simulink model "IndirectFOCControl"  (R2022b)
settings: Solver=VariableStepAuto  StartTime=0.0  StopTime=1  RelTol=1e-3
InitFcn:
  | Data
values from neighbouring files (symbols this model uses):
  delta = 10e-3    (= 0.01)    [Data.m]
  p = 6    [Data.m]    (also in FOC_BANG_Script.m; IFOCdatav6.m)
  Tr = Lm*(1+sigma_r)/Rr    [FOC_BANG_Script.m]    (also in IFOCdatav6.m)
  Vdc = 350    [Data.m]    (also in FOC_BANG_Script.m; IFOCdatav6.m)
libraries: spsControlledVoltageSourceLib x3, spsCurrentMeasurementLib x3, spsAsynchronousMachineSIUnitsLib x1, slpidlib x1, spspowerguiLib x1
settings Model: Creator=v4pal  LastModifiedBy=v4pal

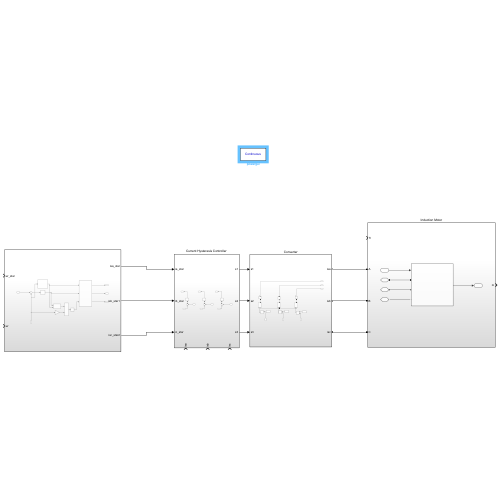
[thumbnail: Simulink's stored preview of the top-level diagram]
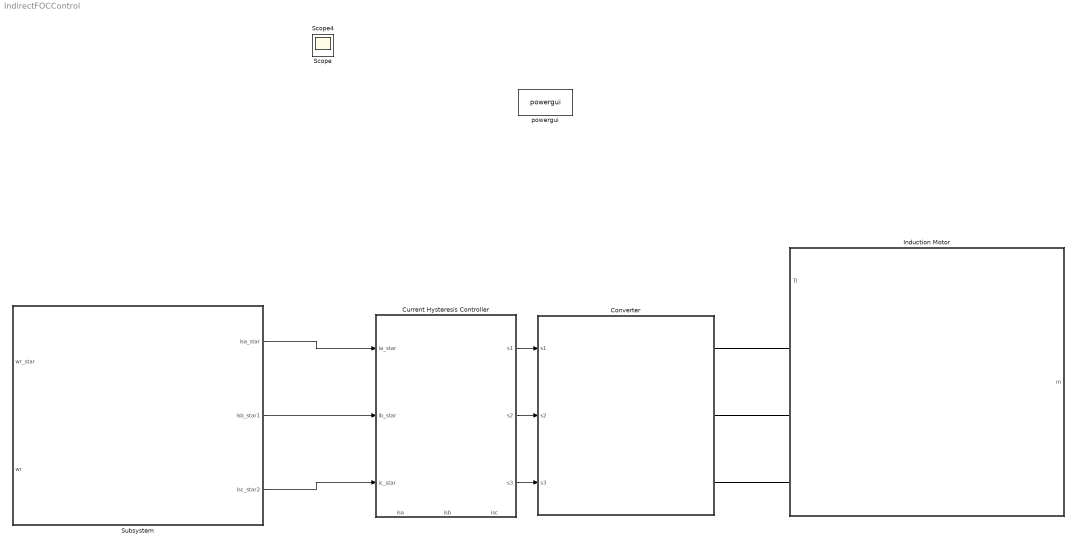
== system IndirectFOCControl ==
  Converter : Subsystem
  "Current Hysteresis Controller " : Subsystem
      settings: PortSchema="{\"entries\":[{\"content\":{\"sides\":[{\"content\":{\"connectorIds\":[\"In1\",\"In2\",\"In3\"]},\"type\":\"ConnectorPlacement.EquallySpacedRectSide\",\"uuid\":\"0262a758-344e-4b59-aa8e-2379075e1762\"},{\"content\":{\"connectorIds\":[\"Out1\",\"Out2\",\"Out3\"],\"side\":\"RIGHT\"},\"type\":\"ConnectorPlacement.EquallySpacedRectSide\",\"uuid\":\"0941517e-4382-4a35-83ac-77ea733cd1ec\"},{\"content\":{\"connectorIds\":[],\"side\":\"TOP\"},\"type\":\"ConnectorPlacement.EquallySpacedRectSide\",\"uuid\":\"ef1a3383-760d-4746-8858-884eb9913812\"},{\"content\":{\"connectorIds\":[\"In4\",\"In5\",\"In6\"],\"side\":\"BOTTOM\"},\"type\":\"ConnectorPlacement.EquallySpacedRectSide\",\"uuid\":\"40fa37ed-c9f4-4172-881b-821ac55ca797\"}]},\"type\":\"ConnectorPlacement.EquallySpacedConnector\",\"uuid\":\"06b611ca-38e4-4d8c-842f-a6960a505aa4\"}],\"packageUris\":[\"http://schema.mathworks.com/mf0/Connector/R2020b\"],\"version\":\"1.0\"}"
  Induction Motor : Subsystem
  Subsystem : Subsystem
  powergui : spspowerguiLib/powergui  Priority=1  SimulationMode=Continuous  SampleTime=50e-6  frequency=60  Iterations=50  frequencyindice=0  Pbase=100e6  ErrMax=1e-4  UnitsV=kV  UnitsW=MW  buscounter=0  FunctionMessages=off  echomessages=off  EnableUseOfTLC=off  CurrentSourceSwitches=off  DisableSnubberDevices=off  DisableRonSwitches=off  DisableVfSwitches=off  DisplayEquations=off  AutomaticDiscreteSolvers=off  SolverType=Tustin/Backward Euler (TBE)  Interpol=off  ExternalGateDelay=off  methode=off  Ts=100  x0status=blocks  SPID=on  SwTol=0  HookPort=off  NonlinearTolerance=1e-4  nMaxIteration=100  ContinueOnMaxIteration=off  RestoreLinks=warning  ResistiveCurrentMeasurement=off  Frange=[0:2:500]  Ylog=off  Xlog=on  ShowGrid=off  save=off  variable=ZData  structure=0  ZoomFFT=off  StartTime=0.0  cycles=1  DisplayStyle=1  fundamental=60  FreqAxis=off  MaxFrequency=1000  frequencyindicesteady=1  RmsSteady=1  display=off
  Scope : Scope
  Scope4 : Scope
  wires:
  "Current Hysteresis Controller "/1(s1) -> Converter/1(s1)
  "Current Hysteresis Controller "/2(s2) -> Converter/2(s2)
  "Current Hysteresis Controller "/3(s3) -> Converter/3(s3)
  Subsystem/1(isa_star) -> "Current Hysteresis Controller "/1(ia_star)
  Subsystem/2(isb_star1) -> "Current Hysteresis Controller "/2(ib_star)
  Subsystem/3(isc_star2) -> "Current Hysteresis Controller "/3(ic_star)
  connections:
  Induction Motor/LConn1 -- Converter/RConn1
  Converter/RConn2 -- Induction Motor/LConn2
  Induction Motor/LConn3 -- Converter/RConn3

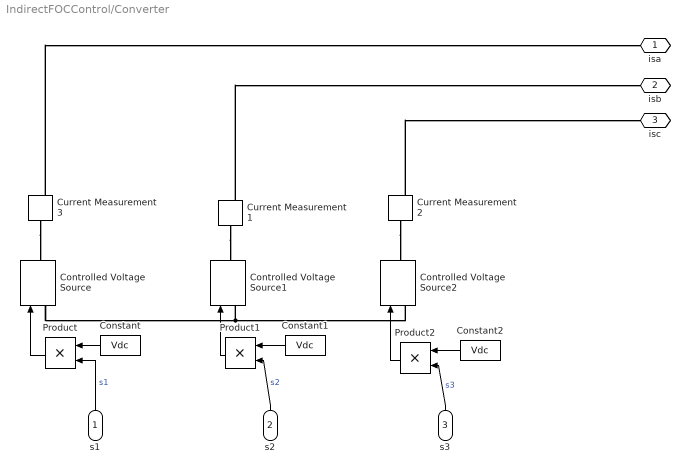
== system IndirectFOCControl/Converter ==
  s1 : Inport
  s2 : Inport  Port=2
  s3 : Inport  Port=3
  Constant : Constant  Value=Vdc
  Constant1 : Constant  Value=Vdc
  Constant2 : Constant  Value=Vdc
  Controlled Voltage Source : spsControlledVoltageSourceLib/Controlled Voltage Source  Initialize=on  Source_Type=AC  Amplitude=0  Phase=0  Frequency=0  Measurements=None
  Controlled Voltage Source1 : spsControlledVoltageSourceLib/Controlled Voltage Source  Initialize=on  Source_Type=AC  Amplitude=0  Phase=0  Frequency=0  Measurements=None
  Controlled Voltage Source2 : spsControlledVoltageSourceLib/Controlled Voltage Source  Initialize=on  Source_Type=AC  Amplitude=0  Phase=0  Frequency=0  Measurements=None
  Current Measurement1 : spsCurrentMeasurementLib/Current Measurement  PhasorSimulation=off  OutputType=Complex  PSBequivalent=0
  Current Measurement2 : spsCurrentMeasurementLib/Current Measurement  PhasorSimulation=off  OutputType=Complex  PSBequivalent=0
  Current Measurement3 : spsCurrentMeasurementLib/Current Measurement  PhasorSimulation=off  OutputType=Complex  PSBequivalent=0
  Product : Product
  Product1 : Product
  Product2 : Product
  isa : PMIOPort  Side=Right
  isb : PMIOPort  Port=2  Side=Right
  isc : PMIOPort  Port=3  Side=Right
  wires:
  Product2/1 -> Controlled Voltage Source2/1
  Constant2/1 -> Product2/1
  Constant/1 -> Product/1
  Product1/1 -> Controlled Voltage Source1/1
  Product/1 -> Controlled Voltage Source/1
  Constant1/1 -> Product1/1
  s2/1 -> Product1/2  "s2"
  s1/1 -> Product/2  "s1"
  s3/1 -> Product2/2  "s3"
  connections:
  Current Measurement1/LConn1 -- Controlled Voltage Source1/RConn1
  Controlled Voltage Source/LConn1 -- Controlled Voltage Source2/LConn1 -- Controlled Voltage Source1/LConn1
  Current Measurement3/LConn1 -- Controlled Voltage Source/RConn1
  Current Measurement2/RConn1 -- isc/RConn1
  Current Measurement2/LConn1 -- Controlled Voltage Source2/RConn1
  Current Measurement1/RConn1 -- isb/RConn1
  Current Measurement3/RConn1 -- isa/RConn1

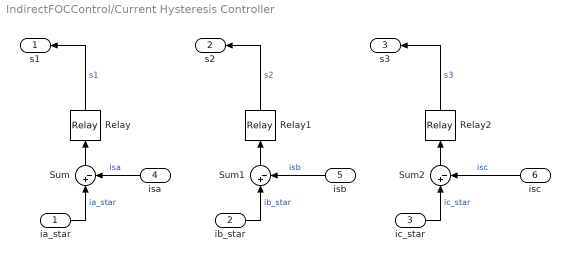
== system IndirectFOCControl/Current Hysteresis Controller  ==
  ia_star : Inport
  ib_star : Inport  Port=2
  ic_star : Inport  Port=3
  isa : Inport  Port=4
  isb : Inport  Port=5
  isc : Inport  Port=6
  Relay : Relay  OnSwitchValue=delta  OffSwitchValue=0
  Relay1 : Relay  OnSwitchValue=delta  OffSwitchValue=0
  Relay2 : Relay  OnSwitchValue=delta  OffSwitchValue=0
  Sum : Sum  Inputs=|+-
  Sum1 : Sum  Inputs=|+-
  Sum2 : Sum  Inputs=|+-
  s1 : Outport
  s2 : Outport  Port=2
  s3 : Outport  Port=3
  wires:
  Sum/1 -> Relay/1
  Sum2/1 -> Relay2/1
  ia_star/1 -> Sum/1  "ia_star"
  isc/1 -> Sum2/2  "isc"
  ic_star/1 -> Sum2/1  "ic_star"
  isa/1 -> Sum/2  "isa"
  Sum1/1 -> Relay1/1
  ib_star/1 -> Sum1/1  "ib_star"
  isb/1 -> Sum1/2  "isb"
  Relay2/1 -> s3/1  "s3"
  Relay/1 -> s1/1  "s1"
  Relay1/1 -> s2/1  "s2"

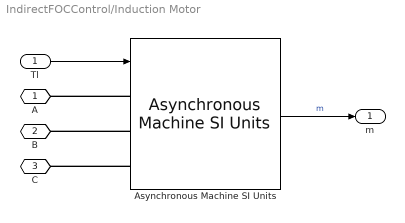
== system IndirectFOCControl/Induction Motor ==
  Tl : Inport
  Asynchronous Machine SI Units : spsAsynchronousMachineSIUnitsLib/Asynchronous Machine SI Units  RotorType=Squirrel-cage  PresetModel=No  MechanicalLoad=Torque Tm  ShowDetailedParameters=on  ReferenceFrame=Rotor  Units=SI  MeasurementBus=off  NominalParameters=[1.845e+04 400 50]  VoltageRatio=1  Stator=[0.5968 0.0003495]  Rotor=[0.6258 0.005473]  Cage1=[0.4155 0.002066]  Cage2=[0.4168 0.0003495]  Lm=0.0354  Mechanical=[0.05 0.005879 2]  PolePairs=2  InitialConditions=[0 0 0 0 0 0 0 0]  SimulateSaturation=off  Saturation=[14.03593122, 27.81365428, 53.79336849, 72.68890987, 97.98006896, 148.6815601, 215.7428561, 302.9841135, 428.7778367 ; 230, 322, 414, 460, 506, 552, 598, 644, 690]  LoadFlowParameters=1492000  TsPowergui=0  TsBlock=-1  IterativeModel=Trapezoidal non iterative  IterativeDiscreteModel=Trapezoidal non iterative  Pmec=1.492e+006
  A : PMIOPort  Side=Left
  B : PMIOPort  Port=2  Side=Left
  C : PMIOPort  Port=3  Side=Left
  m : Outport
  wires:
  Tl/1 -> Asynchronous Machine SI Units/1
  Asynchronous Machine SI Units/1 -> m/1  "m"
  connections:
  Asynchronous Machine SI Units/LConn3 -- C/RConn1
  Asynchronous Machine SI Units/LConn2 -- B/RConn1
  Asynchronous Machine SI Units/LConn1 -- A/RConn1

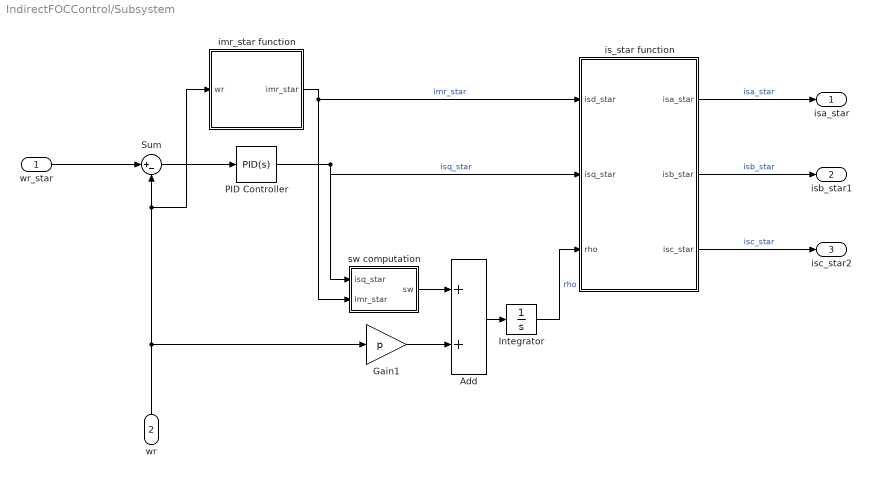
== system IndirectFOCControl/Subsystem ==
  wr_star : Inport
  wr : Inport  Port=2
  Add : Sum
  Gain1 : Gain  Gain=p
  Integrator : Integrator
  PID Controller : slpidlib/PID Controller  Controller=PID  Form=Parallel  TimeDomain=Continuous-time  UseExternalTs=off  SampleTime=-1  IntegratorMethod=Forward Euler  FilterMethod=Forward Euler  ControllerParametersSource=internal  P=1  I=1  UseKiTs=off  D=0  N=100  UseFilter=on  TunerSelectOption=Transfer Function Based (PID Tuner App)  InitialConditionSource=internal  InitialConditionForIntegrator=0  InitialConditionForFilter=0  DifferentiatorICPrevScaledInput=0  ExternalReset=none  TrackingMode=off  Kt=1  LimitOutput=off  SatLimitsSource=internal  UpperSaturationLimit=inf  LowerSaturationLimit=-inf  LinearizeAsGain=on  AntiWindupMode=none  Kb=1  LimitIntegrator=off  UpperIntegratorSaturationLimit=inf  LowerIntegratorSaturationLimit=-inf  POutMin=[]  POutMax=[]  IOutMin=[]  IOutMax=[]  DOutMin=[]  DOutMax=[]  NOutMin=[]  NOutMax=[]  SumOutMin=[]  SumOutMax=[]  SaturationOutMin=[]  SaturationOutMax=[]  PParamMin=[]  PParamMax=[]  IParamMin=[]  IParamMax=[]  DParamMin=[]  DParamMax=[]  NParamMin=[]  NParamMax=[]  KbParamMin=[]  KbParamMax=[]  KtParamMin=[]  KtParamMax=[]  KbOutMin=[]  KbOutMax=[]  KtOutMin=[]  KtOutMax=[]  IntegratorOutMin=[]  IntegratorOutMax=[]  FilterOutMin=[]  FilterOutMax=[]  SumI1OutMin=[]  SumI1OutMax=[]  SumI2OutMin=[]  SumI2OutMax=[]  SumI3OutMin=[]  SumI3OutMax=[]  SumI4OutMin=[]  SumI4OutMax=[]  SumDOutMin=[]  SumDOutMax=[]  DifferentiatorOutMin=[]  DifferentiatorOutMax=[]  FilterDiffOutCoefMin=[]  FilterDiffOutCoefMax=[]  ReciprocalOutMin=[]  ReciprocalOutMax=[]  SumDenOutMin=[]  SumDenOutMax=[]  SumNumOutMin=[]  SumNumOutMax=[]  DivideOutMin=[]  DivideOutMax=[]  UdiffTsProdOutMin=[]  UdiffTsProdOutMax=[]  NTsProdOutMin=[]  NTsProdOutMax=[]  UintegralTsProdOutMin=[]  UintegralTsProdOutMax=[]  UngainTsProdOutMin=[]  UngainTsProdOutMax=[]  ClampingZeroOutDataTypeStr=Inherit: Inherit via back propagation  ClampingZeroOutMin=[]  ClampingZeroOutMax=[]  FilterDenConstantOutDataTypeStr=Inherit: Inherit via back propagation  FilterDenConstantOutMin=[]  FilterDenConstantOutMax=[]  PCopyOutDataTypeStr=Inherit: Inherit via back propagation  PCopyOutMin=[]  PCopyOutMax=[]  NCopyOutDataTypeStr=Inherit: Inherit via back propagation  NCopyOutMin=[]  NCopyOutMax=[]  IntegratorContinuousStateAttributes=''  IntegratorStateMustResolveToSignalObject=off  IntegratorRTWStateStorageClass=Auto  FilterContinuousStateAttributes=''  FilterStateMustResolveToSignalObject=off  FilterRTWStateStorageClass=Auto  ParallelPVariant=InternalParameters  IdealPVariant=Disabled  IVariant=InternalParameters  DVariant=InternalParameters  IntegratorVariant=Continuous  SatVariant=Disabled  AWVariant=Passthrough  PCopyVariant=Disabled  TRVariant=Disabled  FdbkBlocksVariant=Forward  IdealPFdbkVariant=Disabled  SatFdbkVariant=Disabled  DerivativeFilterVariant=ContFilter  NVariant=InternalParameters  NCopyVariant=Disabled  FilterICVariant=InternalICsFilter  IntegratorICVariant=InternalICs  ExternalResetVariant=Disabled  TRSumVariant=Passthrough  SumFdbkVariant=Disabled  SumVariant=Sum_PID  TsampFilterVariant=InternalTs  TsampNgainVariant=Passthrough  TsampIntegralVariant=Passthrough  ExternalSaturationOutDataTypeStr=Inherit: Same as second input
  Sum : Sum  Inputs=|+-
  imr_star function : MATLAB Function  TreatAsAtomicUnit=on
  is_star function : MATLAB Function  TreatAsAtomicUnit=on
  sw computation : Subsystem
  isa_star : Outport
  isb_star1 : Outport  Port=2
  isc_star2 : Outport  Port=3
  wires:
  Integrator/1 -> is_star function/3(rho)  "rho"
  imr_star function/1(imr_star) -> sw computation/2(imr_star), is_star function/1(isd_star)  "imr_star"
  Gain1/1 -> Add/2
  wr/1 -> imr_star function/1(wr), Sum/2, Gain1/1
  Sum/1 -> PID Controller/1
  Add/1 -> Integrator/1
  PID Controller/1 -> sw computation/1(isq_star), is_star function/2(isq_star)  "isq_star"
  sw computation/1(sw) -> Add/1
  wr_star/1 -> Sum/1
  is_star function/1(isa_star) -> isa_star/1  "isa_star"
  is_star function/2(isb_star) -> isb_star1/1  "isb_star"
  is_star function/3(isc_star) -> isc_star2/1  "isc_star"

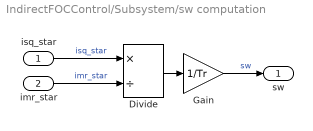
== system IndirectFOCControl/Subsystem/sw computation ==
  isq_star : Inport
  imr_star : Inport  Port=2
  Divide : Product  Inputs=*/  RndMeth=Zero  SaturateOnIntegerOverflow=on
  Gain : Gain  Gain=1/Tr
  sw : Outport
  wires:
  imr_star/1 -> Divide/2  "imr_star"
  Gain/1 -> sw/1  "sw"
  Divide/1 -> Gain/1
  isq_star/1 -> Divide/1  "isq_star"

== matlab function IndirectFOCControl/Subsystem/is_star function ==
  data: isd_star input; isa_star output; isq_star input; rho input; isb_star output; isc_star output
function [isa_star,isb_star, isc_star] = fcn(isd_star, isq_star, rho)

== matlab function IndirectFOCControl/Subsystem/imr_star function ==
  data: wr input; imr_star output
function imr_star = fcn(wr)
